simulink model "ABSv10_01"  (R2020b)
settings: Solver=VariableStepAuto  StartTime=0.0  StopTime=50  RelTol=1e-3
values from neighbouring files (symbols this model uses):
  c1 = 1.2801    [input_1.m]
  c2 = 23.99    [input_1.m]
  c3 = 0.52    [input_1.m]
  c4 = 0.03    [input_1.m]
  fn = m*9.81    (= 3355.02)    [input_1.m]
  jw = 1.13    [input_1.m]
  m = 342    [input_1.m]
  r = 0.33    [input_1.m]
libraries: pid_lib x1
settings Model: Creator=K E S SRINIVAS  LastModifiedBy=Sunny

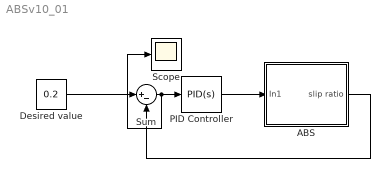
== system ABSv10_01 ==
  ABS : Subsystem
  Desired value : Constant  Value=0.2
  PID Controller : pid_lib/PID Controller  Controller=PID  Form=Parallel  TimeDomain=Continuous-time  UseExternalTs=off  SampleTime=-1  IntegratorMethod=Forward Euler  FilterMethod=Forward Euler  ControllerParametersSource=internal  P=25000  I=1000000  D=10  UseFilter=on  N=100  TunerSelectOption=Transfer Function Based (PID Tuner App)  InitialConditionSource=internal  InitialConditionForIntegrator=0  InitialConditionForFilter=0  DifferentiatorICPrevScaledInput=0  ExternalReset=none  TrackingMode=off  Kt=1  LimitOutput=off  SatLimitsSource=internal  UpperSaturationLimit=inf  LowerSaturationLimit=-inf  LinearizeAsGain=on  AntiWindupMode=none  Kb=1  POutMin=[]  POutMax=[]  IOutMin=[]  IOutMax=[]  DOutMin=[]  DOutMax=[]  NOutMin=[]  NOutMax=[]  SumOutMin=[]  SumOutMax=[]  SaturationOutMin=[]  SaturationOutMax=[]  PParamMin=[]  PParamMax=[]  IParamMin=[]  IParamMax=[]  DParamMin=[]  DParamMax=[]  NParamMin=[]  NParamMax=[]  KbParamMin=[]  KbParamMax=[]  KtParamMin=[]  KtParamMax=[]  KbOutMin=[]  KbOutMax=[]  KtOutMin=[]  KtOutMax=[]  IntegratorOutMin=[]  IntegratorOutMax=[]  FilterOutMin=[]  FilterOutMax=[]  SumI1OutMin=[]  SumI1OutMax=[]  SumI2OutMin=[]  SumI2OutMax=[]  SumI3OutMin=[]  SumI3OutMax=[]  SumI4OutMin=[]  SumI4OutMax=[]  SumDOutMin=[]  SumDOutMax=[]  DifferentiatorOutMin=[]  DifferentiatorOutMax=[]  FilterDiffOutCoefMin=[]  FilterDiffOutCoefMax=[]  ReciprocalOutMin=[]  ReciprocalOutMax=[]  SumDenOutMin=[]  SumDenOutMax=[]  SumNumOutMin=[]  SumNumOutMax=[]  DivideOutMin=[]  DivideOutMax=[]  UdiffTsProdOutMin=[]  UdiffTsProdOutMax=[]  NTsProdOutMin=[]  NTsProdOutMax=[]  UintegralTsProdOutMin=[]  UintegralTsProdOutMax=[]  UngainTsProdOutMin=[]  UngainTsProdOutMax=[]  IntegratorContinuousStateAttributes=''  IntegratorStateMustResolveToSignalObject=off  IntegratorRTWStateStorageClass=Auto  FilterContinuousStateAttributes=''  FilterStateMustResolveToSignalObject=off  FilterRTWStateStorageClass=Auto  ParallelPVariant=InternalParameters  IdealPVariant=Disabled  IVariant=InternalParameters  DVariant=InternalParameters  IntegratorVariant=Continuous  SatVariant=Disabled  AWVariant=Passthrough  PCopyVariant=Disabled  TRVariant=Disabled  FdbkBlocksVariant=Forward  IdealPFdbkVariant=Disabled  SatFdbkVariant=Disabled  DerivativeFilterVariant=ContFilter  NVariant=InternalParameters  NCopyVariant=Disabled  FilterICVariant=InternalICsFilter  IntegratorICVariant=InternalICs  ExternalResetVariant=Disabled  TRSumVariant=Passthrough  SumFdbkVariant=Disabled  SumVariant=Sum_PID  TsampFilterVariant=InternalTs  TsampNgainVariant=Passthrough  TsampIntegralVariant=Passthrough  ExternalSaturationOutDataTypeStr=Inherit: Same as second input
  Scope : Scope
  Sum : Sum  Inputs=|+-
  wires:
  ABS/1(slip ratio) -> Sum/2
  Desired value/1 -> Sum/1
  PID Controller/1 -> ABS/1(In1)
  Sum/1 -> Scope/1, PID Controller/1

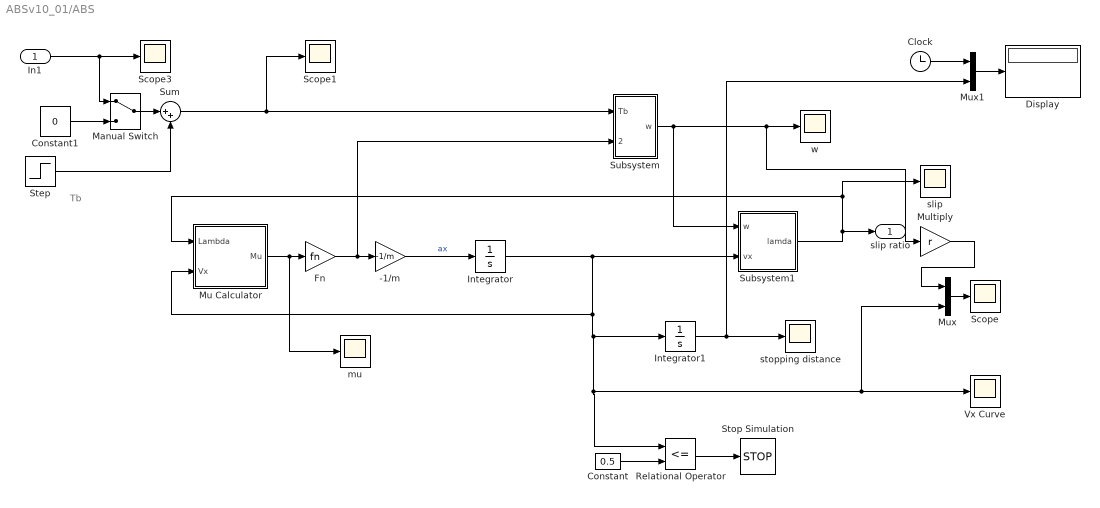
== system ABSv10_01/ABS ==
  note: Tb
  In1 : Inport
  -1/m : Gain  Gain=-1/m
  Clock : Clock
  Constant : Constant  Value=0.5
  Constant1 : Constant  Value=0
  Display : Display
  Fn : Gain  Gain=fn
  Integrator : Integrator  InitialCondition=27.78  LimitOutput=on  LowerSaturationLimit=0
  Integrator1 : Integrator
  Manual Switch : ManualSwitch
  Mu Calculator : Subsystem
  Multiply : Gain  Gain=r
  Mux : Mux  Inputs=2
  Mux1 : Mux  Inputs=2
  Relational Operator : RelationalOperator  Operator=<=  OutDataTypeStr=boolean  RndMeth=Simplest
  Scope : Scope
  Scope1 : Scope
  Scope3 : Scope
  Step : Step  Time=0  After=1200  SampleTime=0
  Stop Simulation : Stop
  Subsystem : Subsystem
  Subsystem1 : Subsystem
  Sum : Sum  Inputs=|++
  Vx Curve : Scope
  mu : Scope
  slip : Scope
  stopping distance : Scope
  w : Scope
  slip ratio : Outport
  wires:
  Mu Calculator/1(Mu) -> mu/1, Fn/1
  Integrator/1 -> Mux/2, Vx Curve/1, Relational Operator/1, Integrator1/1, Mu Calculator/2(Vx), Subsystem1/2(vx)
  -1/m/1 -> Integrator/1  "ax"
  Relational Operator/1 -> Stop Simulation/1
  Constant/1 -> Relational Operator/2
  Sum/1 -> Scope1/1, Subsystem/1(Tb)
  Fn/1 -> Subsystem/2(mu*Fn), -1/m/1
  In1/1 -> Manual Switch/1, Scope3/1
  Step/1 -> Sum/2
  Subsystem/1(w) -> Multiply/1, w/1, Subsystem1/1(w)
  Subsystem1/1(lamda) -> slip/1, Mu Calculator/1(Lambda), slip ratio/1
  Integrator1/1 -> Mux1/2, stopping distance/1
  Mux/1 -> Scope/1
  Multiply/1 -> Mux/1
  Clock/1 -> Mux1/1
  Mux1/1 -> Display/1
  Constant1/1 -> Manual Switch/2
  Manual Switch/1 -> Sum/1

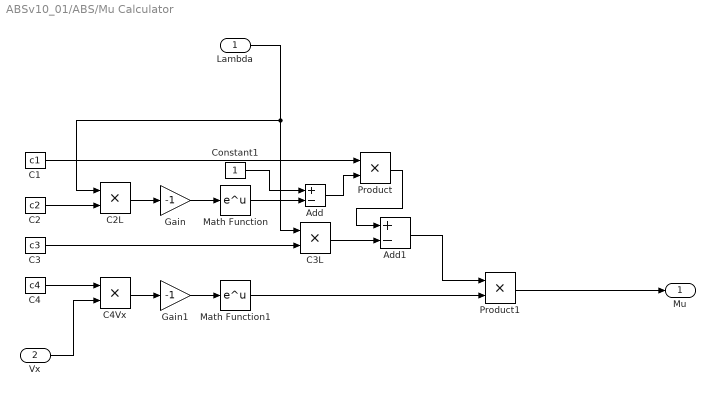
== system ABSv10_01/ABS/Mu Calculator ==
  Lambda : Inport
  Vx : Inport  Port=2
  Add : Sum  Inputs=+-
  Add1 : Sum  Inputs=+-
  C1 : Constant  Value=c1
  C2 : Constant  Value=c2
  C2L : Product
  C3 : Constant  Value=c3
  C3L : Product
  C4 : Constant  Value=c4
  C4Vx : Product
  Constant1 : Constant
  Gain : Gain  Gain=-1
  Gain1 : Gain  Gain=-1
  Math Function : Math  SaturateOnIntegerOverflow=on
  Math Function1 : Math  SaturateOnIntegerOverflow=on
  Product : Product
  Product1 : Product
  Mu : Outport
  wires:
  C2/1 -> C2L/2
  Gain/1 -> Math Function/1
  C1/1 -> Product/1
  C2L/1 -> Gain/1
  Constant1/1 -> Add/1
  Vx/1 -> C4Vx/2
  C4/1 -> C4Vx/1
  Add/1 -> Product/2
  Math Function/1 -> Add/2
  Gain1/1 -> Math Function1/1
  Math Function1/1 -> Product1/2
  C3L/1 -> Add1/2
  Lambda/1 -> C3L/1, C2L/1
  C4Vx/1 -> Gain1/1
  C3/1 -> C3L/2
  Product/1 -> Add1/1
  Add1/1 -> Product1/1
  Product1/1 -> Mu/1

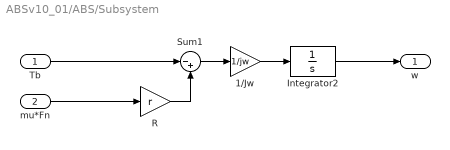
== system ABSv10_01/ABS/Subsystem ==
  Tb : Inport
  mu*Fn : Inport  Port=2
  1/Jw : Gain  Gain=1/jw
  Integrator2 : Integrator  InitialCondition=84.18  LimitOutput=on  LowerSaturationLimit=0
  R : Gain  Gain=r
  Sum1 : Sum  Inputs=|-+
  w : Outport
  wires:
  Sum1/1 -> 1/Jw/1
  Tb/1 -> Sum1/1
  Integrator2/1 -> w/1
  mu*Fn/1 -> R/1
  1/Jw/1 -> Integrator2/1
  R/1 -> Sum1/2

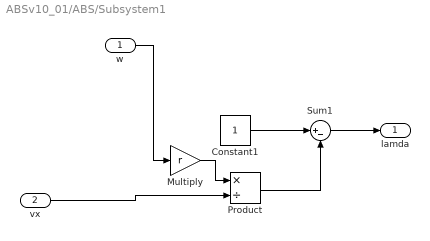
== system ABSv10_01/ABS/Subsystem1 ==
  w : Inport
  vx : Inport  Port=2
  Constant1 : Constant
  Multiply : Gain  Gain=r
  Product : Product  Inputs=*/
  Sum1 : Sum  Inputs=|+-
  lamda : Outport
  wires:
  w/1 -> Multiply/1
  Constant1/1 -> Sum1/1
  vx/1 -> Product/2
  Multiply/1 -> Product/1
  Product/1 -> Sum1/2
  Sum1/1 -> lamda/1
